simulink model "demo_file_13"  (Simulink 8.2)
settings: Solver=ode45  StartTime=0.0  StopTime=100.0  RelTol=1e-3
settings Model: Creator=adokhanc  LastModifiedBy=georgios
settings DataIOCC: SaveFormat=StructureWithTime  SignalLoggingSaveFormat=Dataset
settings OptimizationCC: ExpressionDepthLimit=128
settings DebuggingCC: FcnCallInpInsideContextMsg=EnableAllAsWarning  FrameProcessingCompatibilityMsg=error
settings GRTTargetCC: CodeReplacementLibrary=C89/C90 (ANSI)  CombineOutputUpdateFcns=on  GRTInterface=off

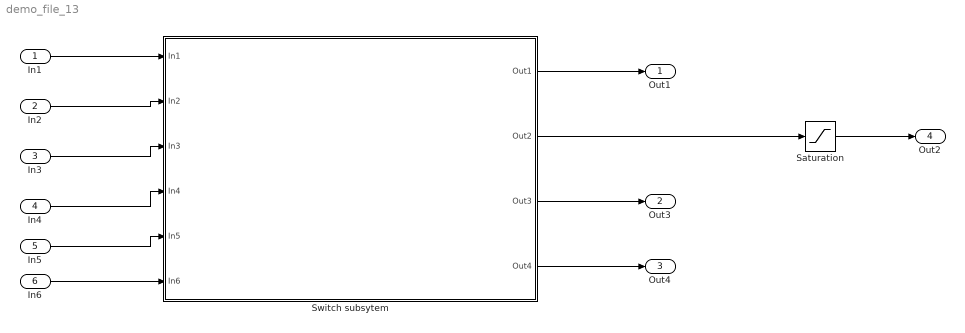
== system demo_file_13 ==
  In1 : Inport
  In2 : Inport  Port=2
  In3 : Inport  Port=3
  In4 : Inport  Port=4
  In5 : Inport  Port=5
  In6 : Inport  Port=6
  Saturation : Saturate  UpperLimit=1  LowerLimit=0.001
  Switch subsytem : Subsystem
  Out1 : Outport
  Out3 : Outport  Port=2
  Out4 : Outport  Port=3
  Out2 : Outport  Port=4
  wires:
  In1/1 -> Switch subsytem/1(In1)
  In2/1 -> Switch subsytem/2(In2)
  In3/1 -> Switch subsytem/3(In3)
  Switch subsytem/2(Out2) -> Saturation/1
  Switch subsytem/1(Out1) -> Out1/1
  Switch subsytem/3(Out3) -> Out3/1
  Switch subsytem/4(Out4) -> Out4/1
  In4/1 -> Switch subsytem/4(In4)
  In5/1 -> Switch subsytem/5(In5)
  In6/1 -> Switch subsytem/6(In6)
  Saturation/1 -> Out2/1

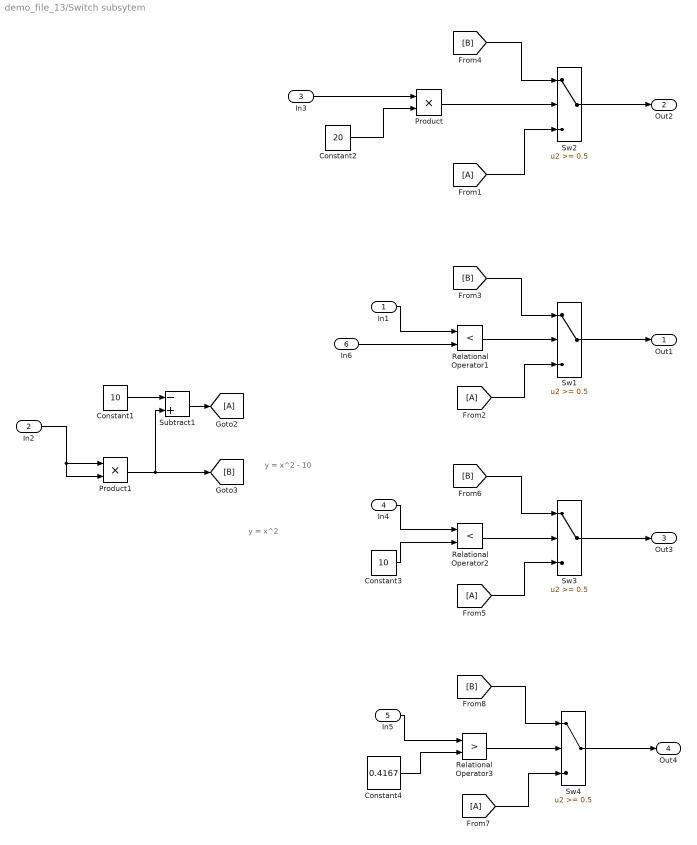
== system demo_file_13/Switch subsytem ==
  note: y = x^2
  note: y = x^2 - 10
  In1 : Inport
  In2 : Inport  Port=2
  In3 : Inport  Port=3
  In4 : Inport  Port=4
  In5 : Inport  Port=5
  In6 : Inport  Port=6
  Constant1 : Constant  Value=10
  Constant2 : Constant  Value=20
  Constant3 : Constant  Value=10
  Constant4 : Constant  Value=0.4167
  Product : Product
  Product1 : Product  RndMeth=Zero
  Relational Operator1 : RelationalOperator  Operator=<  OutDataTypeStr=boolean
  Relational Operator2 : RelationalOperator  Operator=<  OutDataTypeStr=boolean
  Relational Operator3 : RelationalOperator  Operator=>  OutDataTypeStr=boolean
  Subtract1 : Sum  Inputs=-+
  Sw{1..4} (4 alike) : Switch  Threshold=0.5  RndMeth=Simplest  InputSameDT=on
  Out1 : Outport
  Out2 : Outport  Port=2
  Out3 : Outport  Port=3
  Out4 : Outport  Port=4
  wires:
  In6/1 -> Relational Operator1/2
  Relational Operator1/1 -> Sw1/2
  Product1/1 -> Subtract1/2, [B]
  Constant1/1 -> Subtract1/1
  Subtract1/1 -> [A]
  In2/1 -> Product1/2, Product1/1
  [A] -> Sw1/3
  [B] -> Sw1/1
  Sw1/1 -> Out1/1
  [A] -> Sw2/3
  [B] -> Sw2/1
  Sw2/1 -> Out2/1
  In3/1 -> Product/1
  Constant2/1 -> Product/2
  Product/1 -> Sw2/2
  In4/1 -> Relational Operator2/1
  Constant3/1 -> Relational Operator2/2
  Relational Operator2/1 -> Sw3/2
  [A] -> Sw3/3
  [B] -> Sw3/1
  Sw3/1 -> Out3/1
  In5/1 -> Relational Operator3/1
  Constant4/1 -> Relational Operator3/2
  Relational Operator3/1 -> Sw4/2
  [A] -> Sw4/3
  [B] -> Sw4/1
  Sw4/1 -> Out4/1
  In1/1 -> Relational Operator1/1
